simulink model "inverter_APF"  (R2013b)
settings: Solver=ode23t  StartTime=0.0  StopTime=0.3  RelTol=1e-3
StopFcn:
  | T= ScopeData.time;
  | V_DC= ScopeData.signals(1,1).values;
  | V_LL=ScopeData2.signals.values;
  | subplot(2,1,1);
  | plot(T,V_LL);title('Line to Line Voltage Vab','fontsize',16);xlabel('t');ylabel('V');grid on;
  | subplot(2,1,2);
  | plot(T,V_DC);title('DC link Voltage Vdc','fontsize',16);xlabel('t');ylabel('V');grid on;
libraries: powerlib x17, powerlib_extras x1
settings Model: Creator=sample  LastModifiedBy=kasth
settings DataIOCC: SignalLoggingSaveFormat=ModelDataLogs
settings OptimizationCC: ExpressionDepthLimit=2147483647
settings DebuggingCC: FcnCallInpInsideContextMsg=EnableAllAsWarning  StateNameClashWarn=warning
settings GRTTargetCC: CombineOutputUpdateFcns=off  GRTInterface=on

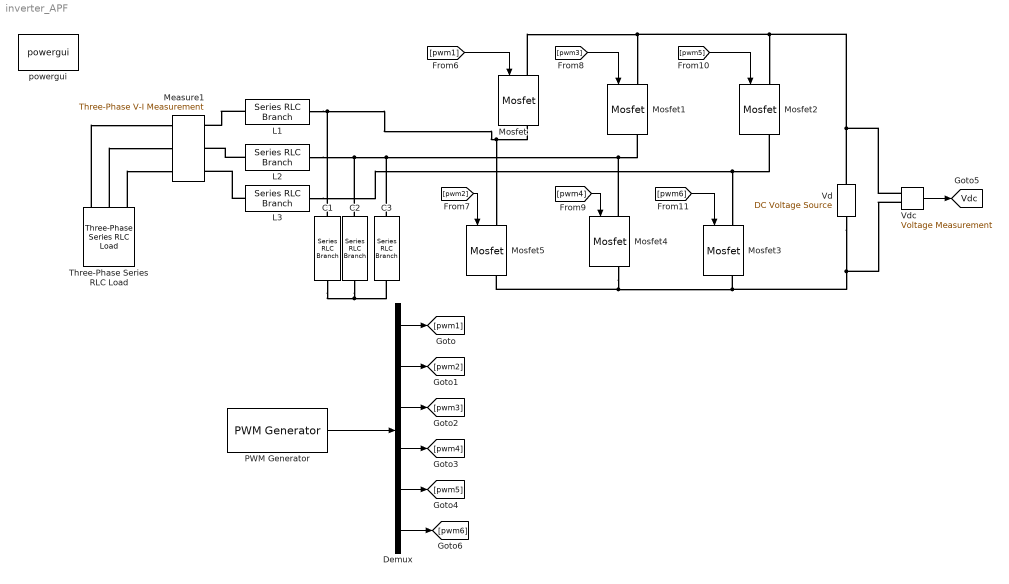
== system inverter_APF ==
  C1 : powerlib/Elements/Series RLC Branch  LConnTagsString=__new0  RConnTagsString=__new0  BranchType=C  Resistance=1  Inductance=18e-3  SetiL0=off  InitialCurrent=0  Capacitance=80e-6  Setx0=off  InitialVoltage=0  Measurements=None
  C2 : powerlib/Elements/Series RLC Branch  LConnTagsString=__new0  RConnTagsString=__new0  BranchType=C  Resistance=1  Inductance=18e-3  SetiL0=off  InitialCurrent=0  Capacitance=80e-6  Setx0=off  InitialVoltage=0  Measurements=None
  C3 : powerlib/Elements/Series RLC Branch  LConnTagsString=__new0  RConnTagsString=__new0  BranchType=C  Resistance=1  Inductance=18e-3  SetiL0=off  InitialCurrent=0  Capacitance=80e-6  Setx0=off  InitialVoltage=0  Measurements=None
  Demux : Demux  Outputs=6
  L1 : powerlib/Elements/Series RLC Branch  LConnTagsString=__new0  RConnTagsString=__new0  BranchType=L  Resistance=1  Inductance=18e-3  SetiL0=off  InitialCurrent=0  Capacitance=1e-6  Setx0=off  InitialVoltage=0  Measurements=None
  L2 : powerlib/Elements/Series RLC Branch  LConnTagsString=__new0  RConnTagsString=__new0  BranchType=L  Resistance=1  Inductance=18e-3  SetiL0=off  InitialCurrent=0  Capacitance=1e-6  Setx0=off  InitialVoltage=0  Measurements=None
  L3 : powerlib/Elements/Series RLC Branch  LConnTagsString=__new0  RConnTagsString=__new0  BranchType=L  Resistance=1  Inductance=18e-3  SetiL0=off  InitialCurrent=0  Capacitance=1e-6  Setx0=off  InitialVoltage=0  Measurements=None
  Measure1 : powerlib/Measurements/Three-Phase V-I Measurement  VoltageMeasurement=phase-to-phase  SetLabelV=on  LabelV=Vabc_load  Vpu=off  VpuLL=off  CurrentMeasurement=yes  SetLabelI=on  LabelI=I1  Ipu=off  Pbase=1e3  Vbase=380  OutputType=Magnitude  PhasorSimulation=off  PSBequivalent=0
  Mosfet{,1..5} (6 alike) : powerlib/Power Electronics/Mosfet  Ron=0.1  Lon=0  Rd=0.01  Vfd=0  IC=0  Rs=1e5  Cs=inf  Measurements=on
  PWM Generator : powerlib_extras/Control  Blocks/PWM Generator  GeneratorMode="3-arm  bridge (6 pulses)"  Fc=2e3  Internal=on  mIndex=1  Freq=50  Phase=0
  Three-Phase Series RLC Load : powerlib/Elements/Three-Phase Series RLC Load  LConnTagsString=A|B|C  Configuration=Y (grounded)  NominalVoltage=1000  NominalFrequency=60  ActivePower=10e3  InductivePower=100  CapacitivePower=100  Measurements=None  LoadType=constant Z
  Vd : powerlib/Electrical Sources/DC Voltage Source  Amplitude=700  Measurements=None
  "Vdc " : powerlib/Measurements/Voltage Measurement  Tag=PoWeRsYsTeMmEaSuReMeNt  PhasorSimulation=off  OutputType=Magnitude  PSBequivalent=0
  powergui : powerlib/powergui  Priority=1  SimulationMode=Discrete  SolverType=Tustin  SampleTime=50e-6  frequency=60  SPID=off  DisableSnubberDevices=off  DisableRonSwitches=off  DisableVfSwitches=off  SwTol=0  Interpol=off  DisplayEquations=off  frequencyindice=0  Pbase=100e6  ErrMax=1e-4  Iterations=50  UnitsV=kV  UnitsW=MW  FunctionMessages=off  echomessages=off  HookPort=off  EnableUseOfTLC=off  x0status=blocks  RestoreLinks=warning  ResistiveCurrentMeasurement=off  Frange=[0:2:500]  Ylog=off  Xlog=on  ShowGrid=off  save=off  variable=ZData  structure=sourcecurrent  ZoomFFT=off  StartTime=0.01  cycles=1  DisplayStyle=1  fundamental=50  FreqAxis=on  MaxFrequency=1000  frequencyindicesteady=1  RmsSteady=1  display=off  Ts=0  methode=off
  tag scope: Vdc=global
  wires:
  "Vdc "/1 -> [Vdc]
  Demux/1 -> [pwm1]
  Demux/2 -> [pwm2]
  Demux/3 -> [pwm3]
  Demux/4 -> [pwm4]
  Demux/5 -> [pwm5]
  Demux/6 -> [pwm6]
  [pwm1] -> Mosfet/1
  [pwm2] -> Mosfet5/1
  [pwm3] -> Mosfet1/1
  [pwm4] -> Mosfet4/1
  [pwm5] -> Mosfet2/1
  [pwm6] -> Mosfet3/1
  PWM Generator/1 -> Demux/1
  connections:
  Vd/RConn1 -- "Vdc "/LConn1 -- Mosfet/LConn1 -- Mosfet1/LConn1 -- Mosfet2/LConn1
  Mosfet5/RConn1 -- Mosfet4/RConn1 -- "Vdc "/LConn2 -- Vd/LConn1 -- Mosfet3/RConn1
  C1/LConn1 -- L1/RConn1 -- Mosfet5/LConn1 -- Mosfet/RConn1
  L2/RConn1 -- C2/LConn1 -- C3/LConn1 -- Mosfet4/LConn1 -- Mosfet1/RConn1
  L3/RConn1 -- Mosfet3/LConn1 -- Mosfet2/RConn1
  L1/LConn1 -- Measure1/LConn1
  L2/LConn1 -- Measure1/LConn2
  L3/LConn1 -- Measure1/LConn3
  C1/RConn1 -- C2/RConn1 -- C3/RConn1
  Three-Phase Series RLC Load/LConn1 -- Measure1/RConn1
  Three-Phase Series RLC Load/LConn2 -- Measure1/RConn2
  Three-Phase Series RLC Load/LConn3 -- Measure1/RConn3
